simulink model "Simulation_Dual"  (R2022b)
settings: Solver=FixedStepAuto  StartTime=0.0  StopTime=5  FixedStep=1e-6  RelTol=1e-3
model workspace (MAT data in the model file):
  Fbase = 50
  Filter_Ind = 0.00435
  Fs = 10000
  Series1_L = 0.004
  Series2_L = 0.00035
  Shunt_C = 2.2e-06
  Snubber_C = inf
  Snubber_R = 100000
  Ts = 0.0001
  VDCref = 48
undefined symbols (not defined in the file): DiscIntNeverNeededParam, Rdamp, Series1_C, Series2_R
libraries: spsPWMGeneratorDCDCLib x6, spsThreePhaseSeriesRLCBranchLib x6, spsVoltageMeasurementLib x6, spsabctodq0Lib x4, spsThreePhaseVIMeasurementLib x3, spsDCVoltageSourceLib x2, spsdq0toabcLib x2, spsUniversalBridgeLib x2, simulink x1, spspowerguiLib x1
settings Model: Creator=yanni  LastModifiedBy=yanni

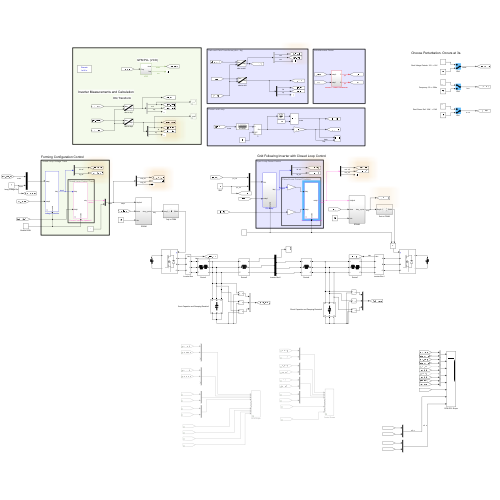
[thumbnail: Simulink's stored preview of the top-level diagram]
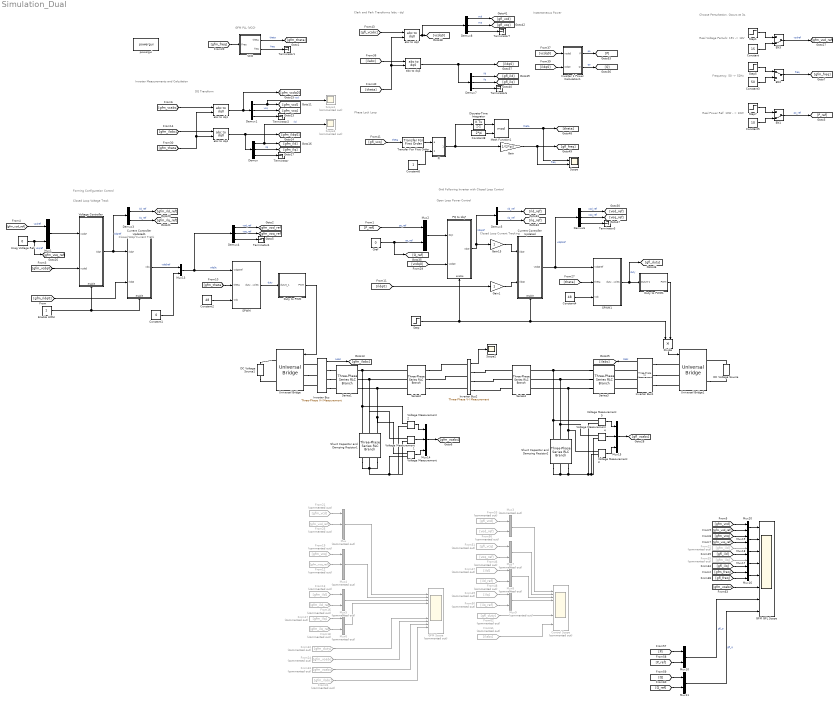
== system Simulation_Dual ==
  note: Closed Loop Voltage Track
  note: Closed Loop Current Track
  note: DQ Transform
  note: GFM PLL (VCO)
  note: Forming Configuration Control
  note: Inverter Measurements and Calculation
  note: Grid Following Inverter with Closed Loop Control
  note: Open Loop Power Control
  note: Closed Loop Current Tracking
  note: Phase Lock Loop
  note: Instantaneous Power
  note: Clark and Park Transforms (abc - dq)
  note: Choose Perturbation. Occurs at 3s.
  note: Real Voltage Perturb: 15V -> 18V
  note: Frequency: 50 -> 52Hz
  note: Real Power Ref: 10W - > 10W
  Constant : Constant  Value=15
  Constant1 : Constant  Value=0
  Constant2 : Constant  Value=48
  Constant3 : Constant  Value=50
  Constant4 : Constant  Value=48
  Constant5 : Constant  Value=10
  Constant6 : Constant
  Constant8 : Constant  Value=2*pi
  Control Scope : Scope  Commented=on  NumInputPorts=12
  Current Controller Updated : Subsystem  mask{Id_Proportional=1.22, Id_Integral=957/16}
      mask prompts: Id_Proportional "Kp"; Id_Integral "Ki"
      settings: PortSchema="{\"entries\":[{\"content\":{\"sides\":[{\"content\":{\"connectorIds\":[\"In1\",\"In2\"]},\"type\":\"ConnectorPlacement.EquallySpacedRectSide\",\"uuid\":\"134caf41-c34b-48d0-a71a-522329c40d8c\"},{\"content\":{\"connectorIds\":[\"Out1\"],\"side\":\"RIGHT\"},\"type\":\"ConnectorPlacement.EquallySpacedRectSide\",\"uuid\":\"de6d8359-09d9-4cb7-8990-bc4b6d48f18d\"},{\"content\":{\"connectorIds\":[],\"side\":\"TOP\"},\"type\":\"ConnectorPlacement.EquallySpacedRectSide\",\"uuid\":\"e2785d07-2ead-4d42-94ac-8025f550e46a\"},{\"content\":{\"connectorIds\":[\"In3\"],\"side\":\"BOTTOM\"},\"type\":\"ConnectorPlacement.EquallySpacedRectSide\",\"uuid\":\"a912a274-012c-4cba-911c-beb79bb7dc91\"}]},\"type\":\"ConnectorPlacement.EquallySpacedConnector\",\"uuid\":\"3c498838-bb9a-4b09-bf48-00f71cabf7b4\"}],\"packageUris\":[\"http://schema.mathworks.com/mf0/Connector/R2020b\"],\"version\":\"1.0\"}"
  Current Controller Updated1 : Subsystem  mask{Id_Proportional=0.61, Id_Integral=240/16}
      mask prompts: Id_Proportional "Kp"; Id_Integral "Ki"
      settings: PortSchema="{\"entries\":[{\"content\":{\"sides\":[{\"content\":{\"connectorIds\":[\"In1\",\"In2\"]},\"type\":\"ConnectorPlacement.EquallySpacedRectSide\",\"uuid\":\"134caf41-c34b-48d0-a71a-522329c40d8c\"},{\"content\":{\"connectorIds\":[\"Out1\"],\"side\":\"RIGHT\"},\"type\":\"ConnectorPlacement.EquallySpacedRectSide\",\"uuid\":\"de6d8359-09d9-4cb7-8990-bc4b6d48f18d\"},{\"content\":{\"connectorIds\":[],\"side\":\"TOP\"},\"type\":\"ConnectorPlacement.EquallySpacedRectSide\",\"uuid\":\"e2785d07-2ead-4d42-94ac-8025f550e46a\"},{\"content\":{\"connectorIds\":[\"In3\"],\"side\":\"BOTTOM\"},\"type\":\"ConnectorPlacement.EquallySpacedRectSide\",\"uuid\":\"a912a274-012c-4cba-911c-beb79bb7dc91\"}]},\"type\":\"ConnectorPlacement.EquallySpacedConnector\",\"uuid\":\"3c498838-bb9a-4b09-bf48-00f71cabf7b4\"}],\"packageUris\":[\"http://schema.mathworks.com/mf0/Connector/R2020b\"],\"version\":\"1.0\"}"
  DC Voltage Source : spsDCVoltageSourceLib/DC Voltage Source  Amplitude=VDCref  Measurements=None
  DC Voltage Source1 : spsDCVoltageSourceLib/DC Voltage Source  Amplitude=48  Measurements=None
  Demux{,1,4,6..8} (6 alike) : Demux  Outputs=3
  Demux3 : Demux  Outputs=2
  Demux5 : Demux  Outputs=2
  Discrete-Time Integrator : DiscreteIntegrator  SampleTime=Ts  ICPrevOutput=DiscIntNeverNeededParam  ICPrevScaledInput=DiscIntNeverNeededParam
  Divide : Product  Inputs=**
  Duty to PWM : Subsystem
  Duty to PWM1 : Subsystem
  EN1 : ManualSwitch  CurrentSetting=0
  EN2 : ManualSwitch
  EN3 : ManualSwitch  CurrentSetting=0
  Enable HIGH : Constant
  From12 : From  Commented=on  GotoTag=gfm_voq_ref
      settings: CloseFcn=tagdialog Close
  From13 : From  Commented=on  GotoTag=gfm_ild
      settings: CloseFcn=tagdialog Close
  From16 : From  Commented=on  GotoTag=gfm_ild_ref
      settings: CloseFcn=tagdialog Close
  From17 : From  Commented=on  GotoTag=gfm_ilq
      settings: CloseFcn=tagdialog Close
  From18 : From  Commented=on  GotoTag=gfm_ilq_ref
      settings: CloseFcn=tagdialog Close
  From19 : From  Commented=on  GotoTag=gfm_vcq
      settings: CloseFcn=tagdialog Close
  From21 : From  Commented=on  GotoTag=gfm_vcd
      settings: CloseFcn=tagdialog Close
  From22 : From  Commented=on  GotoTag=gfm_ild
      settings: CloseFcn=tagdialog Close
  From24 : From  Commented=on  GotoTag=gfm_voabc
      settings: CloseFcn=tagdialog Close
  From25 : From  Commented=on  GotoTag=gfm_vod_ref
      settings: CloseFcn=tagdialog Close
  From31 : From  Commented=on  GotoTag=gfm_ilabc
      settings: CloseFcn=tagdialog Close
  From32 : From  Commented=on  GotoTag=gfm_duty
      settings: CloseFcn=tagdialog Close
  From33 : From  Commented=on  GotoTag=gfm_vcabc
      settings: CloseFcn=tagdialog Close
  From35 : From  Commented=on  GotoTag=gfm_ilq
      settings: CloseFcn=tagdialog Close
  From46 : From  Commented=on  GotoTag=voq_ref
      settings: CloseFcn=tagdialog Close
  From47 : From  Commented=on  GotoTag=ild
      settings: CloseFcn=tagdialog Close
  From48 : From  Commented=on  GotoTag=ild_ref
      settings: CloseFcn=tagdialog Close
  From49 : From  Commented=on  GotoTag=ilq
      settings: CloseFcn=tagdialog Close
  From50 : From  Commented=on  GotoTag=ilq_ref
      settings: CloseFcn=tagdialog Close
  From51 : From  Commented=on  GotoTag=gfl_vcq
      settings: CloseFcn=tagdialog Close
  From53 : From  Commented=on  GotoTag=gfl_vcd
      settings: CloseFcn=tagdialog Close
  From56 : From  Commented=on  GotoTag=vod_ref
      settings: CloseFcn=tagdialog Close
  From61 : From  Commented=on  GotoTag=ilabc
      settings: CloseFcn=tagdialog Close
  From62 : From  Commented=on  GotoTag=gfl_duty
      settings: CloseFcn=tagdialog Close
  GFM GFL Scope : Scope  NumInputPorts=8
  GFM Scope : Scope  Commented=on  NumInputPorts=12
  Gain : Gain  Gain=1/(2*pi)
  Gain1 : Gain
  Gain15 : Gain
  Imag Votlage Ref : Constant  Value=0
  Inverter 1 Power Calculation1 : Subsystem
  Inverter Bus : spsThreePhaseVIMeasurementLib/Three-Phase V-I Measurement  VoltageMeasurement=no  SetLabelV=off  LabelV=Vabc  Vpu=off  VpuLL=off  CurrentMeasurement=yes  SetLabelI=off  LabelI=Iabc  Ipu=off  Pbase=100e6  Vbase=500e3  OutputType=Complex  PhasorSimulation=off  PSBequivalent=0
  Inverter Bus1 : spsThreePhaseVIMeasurementLib/Three-Phase V-I Measurement  VoltageMeasurement=no  SetLabelV=off  LabelV=Vabc  Vpu=off  VpuLL=off  CurrentMeasurement=yes  SetLabelI=off  LabelI=Iabc  Ipu=off  Pbase=100e6  Vbase=500e3  OutputType=Complex  PhasorSimulation=off  PSBequivalent=0
  Inverter Bus2 : spsThreePhaseVIMeasurementLib/Three-Phase V-I Measurement  VoltageMeasurement=phase-to-phase  SetLabelV=off  LabelV=Vabc  Vpu=off  VpuLL=off  CurrentMeasurement=no  SetLabelI=off  LabelI=Iabc  Ipu=off  Pbase=100e6  Vbase=500e3  OutputType=Complex  PhasorSimulation=off  PSBequivalent=0
  Math Function1 : Math  Operator=mod  SignedPower=on
  Mux : Mux  Commented=on  Inputs=3
  Mux{1..2,10..11,13,16..20} (10 alike) : Mux  Inputs=2
  Mux14 : Mux  Inputs=3
  Mux15 : Mux  Inputs=3
  Mux{3,5..9} (6 alike) : Mux  Commented=on  Inputs=2
  Mux4 : Mux  Commented=on  Inputs=3
  PI : Subsystem  mask{Kp_PLL=6.09, Ki_PLL=9.57, IntSat_PLL=20000}
      mask prompts: Kp_PLL "Proportional (P)"; Ki_PLL "Integral (I)"; IntSat_PLL "Integrator Saturation Limit"
      mask DialogControl DescGroupVar Prompt: PLL Parameters
  PQ to Idq* : Subsystem
      settings: PortSchema="{\"entries\":[{\"content\":{\"sides\":[{\"content\":{\"connectorIds\":[\"In1\",\"In2\"]},\"type\":\"ConnectorPlacement.EquallySpacedRectSide\",\"uuid\":\"5271b3ed-46a4-4113-9b69-458d23b85fa2\"},{\"content\":{\"connectorIds\":[\"Out1\"],\"side\":\"RIGHT\"},\"type\":\"ConnectorPlacement.EquallySpacedRectSide\",\"uuid\":\"00fb532b-4b50-4607-a5c4-cd74a5a5fc42\"},{\"content\":{\"connectorIds\":[],\"side\":\"TOP\"},\"type\":\"ConnectorPlacement.EquallySpacedRectSide\",\"uuid\":\"05671b8e-b1fa-45d3-a4a8-1640aa1af326\"},{\"content\":{\"connectorIds\":[\"In3\"],\"side\":\"BOTTOM\"},\"type\":\"ConnectorPlacement.EquallySpacedRectSide\",\"uuid\":\"cfa1ca65-6f63-4245-906b-c8bf76b96ed3\"}]},\"type\":\"ConnectorPlacement.EquallySpacedConnector\",\"uuid\":\"bf062c94-390f-4409-83d1-f8a32d59f496\"}],\"packageUris\":[\"http://schema.mathworks.com/mf0/Connector/R2020b\"],\"version\":\"1.0\"}"
  Qref : Constant  Value=0
  SPWM : Subsystem
  SPWM1 : Subsystem
  Scope : Scope  NumInputPorts=2
  Scope1 : Scope  Commented=on
  Scope2 : Scope
  Scope3 : Scope  Commented=on
  Series1 : spsThreePhaseSeriesRLCBranchLib/Three-Phase Series RLC Branch  LConnTagsString=A|B|C  RConnTagsString=A|B|C  BranchType=RL  Resistance=0.35  Inductance=Series1_L  Capacitance=Series1_C  Measurements=None
  Series2 : spsThreePhaseSeriesRLCBranchLib/Three-Phase Series RLC Branch  LConnTagsString=A|B|C  RConnTagsString=A|B|C  BranchType=L  Resistance=Series2_R  Inductance=Series2_L  Capacitance=1e-6  Measurements=None
  Series3 : spsThreePhaseSeriesRLCBranchLib/Three-Phase Series RLC Branch  LConnTagsString=A|B|C  RConnTagsString=A|B|C  BranchType=RL  Resistance=0.35  Inductance=Series1_L  Capacitance=Series1_C  Measurements=None
  Series4 : spsThreePhaseSeriesRLCBranchLib/Three-Phase Series RLC Branch  LConnTagsString=A|B|C  RConnTagsString=A|B|C  BranchType=L  Resistance=Series2_L  Inductance=Series2_L  Capacitance=1e-6  Measurements=None
  Shunt Capacitor and Damping Resistor1 : spsThreePhaseSeriesRLCBranchLib/Three-Phase Series RLC Branch  LConnTagsString=A|B|C  RConnTagsString=A|B|C  BranchType=C  Resistance=Rdamp  Inductance=1e-3  Capacitance=Shunt_C  Measurements=None
  Shunt Capacitor and Damping Resistor2 : spsThreePhaseSeriesRLCBranchLib/Three-Phase Series RLC Branch  LConnTagsString=A|B|C  RConnTagsString=A|B|C  BranchType=C  Resistance=Rdamp  Inductance=1e-3  Capacitance=Shunt_C  Measurements=None
  Step : Step  SampleTime=0
  Step1 : Step  Time=3  Before=15  After=18
  Step5 : Step  Time=3  Before=50  After=52  SampleTime=0
  Step7 : Step  Time=3  Before=10  After=-10
  Terminator{,1..4,6..7} (7 alike) : Terminator
  Transfer Fcn First Order : simulink/Discrete/Transfer Fcn First Order  PoleZ=exp(-2*pi*100*Ts)  ICPrevOutput=0.0  DoSatur=off
  Universal Bridge : spsUniversalBridgeLib/Universal Bridge  Arms=3  SnubberResistance=Snubber_R  SnubberCapacitance=Snubber_C  Device=MOSFET / Diodes  Ron=1e-3  Lon=0  ForwardVoltages="[  0  0  ]"  ForwardVoltage=0  GTOparameters=[ 10e-6 , 20e-6 ]  IGBTparameters=[ 1e-6 , 2e-6 ]  Measurements=None  Measurements_2=None  converterType=Rectifier
  Universal Bridge1 : spsUniversalBridgeLib/Universal Bridge  Arms=3  SnubberResistance=Snubber_R  SnubberCapacitance=Snubber_C  Device=MOSFET / Diodes  Ron=1e-3  Lon=0  ForwardVoltages="[  0  0  ]"  ForwardVoltage=0  GTOparameters=[ 10e-6 , 20e-6 ]  IGBTparameters=[ 1e-6 , 2e-6 ]  Measurements=All voltages and currents  Measurements_2=None  converterType=Rectifier
  VCO : Subsystem
  Voltage Controller : Subsystem  mask{Id_Proportional=0.028, Id_Integral=8.685*8}
      mask prompts: Id_Proportional "Kp"; Id_Integral "Ki"
      settings: PortSchema="{\"entries\":[{\"content\":{\"sides\":[{\"content\":{\"connectorIds\":[\"In1\",\"In2\"]},\"type\":\"ConnectorPlacement.EquallySpacedRectSide\",\"uuid\":\"134caf41-c34b-48d0-a71a-522329c40d8c\"},{\"content\":{\"connectorIds\":[\"Out1\"],\"side\":\"RIGHT\"},\"type\":\"ConnectorPlacement.EquallySpacedRectSide\",\"uuid\":\"de6d8359-09d9-4cb7-8990-bc4b6d48f18d\"},{\"content\":{\"connectorIds\":[],\"side\":\"TOP\"},\"type\":\"ConnectorPlacement.EquallySpacedRectSide\",\"uuid\":\"e2785d07-2ead-4d42-94ac-8025f550e46a\"},{\"content\":{\"connectorIds\":[\"In3\"],\"side\":\"BOTTOM\"},\"type\":\"ConnectorPlacement.EquallySpacedRectSide\",\"uuid\":\"a912a274-012c-4cba-911c-beb79bb7dc91\"}]},\"type\":\"ConnectorPlacement.EquallySpacedConnector\",\"uuid\":\"3c498838-bb9a-4b09-bf48-00f71cabf7b4\"}],\"packageUris\":[\"http://schema.mathworks.com/mf0/Connector/R2020b\"],\"version\":\"1.0\"}"
  Voltage Measurement{,1..5} (6 alike) : spsVoltageMeasurementLib/Voltage Measurement  PhasorSimulation=off  OutputType=Complex  PSBequivalent=0
  abc to dq{1..4} (4 alike) : spsabctodq0Lib/abc to dq0  Alignment=90 degrees behind phase A axis
  powergui : spspowerguiLib/powergui  Priority=1  SimulationMode=Discrete  SampleTime=1e-6  frequency=60  Iterations=50  frequencyindice=0  Pbase=100e6  ErrMax=1e-4  UnitsV=kV  UnitsW=MW  buscounter=0  FunctionMessages=off  echomessages=off  EnableUseOfTLC=off  CurrentSourceSwitches=off  DisableSnubberDevices=off  DisableRonSwitches=off  DisableVfSwitches=off  DisplayEquations=off  AutomaticDiscreteSolvers=off  SolverType=Tustin/Backward Euler (TBE)  Interpol=off  ExternalGateDelay=off  methode=off  Ts=100  x0status=blocks  SPID=on  SwTol=0  HookPort=off  NonlinearTolerance=1e-4  nMaxIteration=100  ContinueOnMaxIteration=off  RestoreLinks=warning  ResistiveCurrentMeasurement=off  Frange=[0:2:500]  Ylog=off  Xlog=on  ShowGrid=off  save=off  variable=ZData  structure=0  ZoomFFT=off  StartTime=0.0  cycles=1  DisplayStyle=1  fundamental=60  FreqAxis=off  MaxFrequency=1000  frequencyindicesteady=1  RmsSteady=1  display=off
  wires:
  abc to dq1/1 -> [gfm_vcdq0], Demux1/1
  Mux13/1 -> SPWM/1(Vdq0ref), Demux4/1  "vdq0c"
  abc to dq4/1 -> [gfm_ildq0], Demux/1
  [gfm_theta] -> SPWM/2(theta)
  Enable HIGH/1 -> Current Controller Updated1/3(enable), Voltage Controller/3(enable)
  Mux1/1 -> Voltage Controller/1(vsdq*)
  [gfm_vsd_ref] -> Mux1/1  "vsdref"
  Imag Votlage Ref/1 -> [gfm_vsq_ref], Mux1/2  "vsqref"
  Inverter Bus/1 -> [gfm_ilabc]  "iLabc"
  Demux/2 -> [gfm_ilq]  "ilq"
  Demux/1 -> Scope3/1, [gfm_ild]  "ild"
  Demux/3 -> Terminator/1
  Demux3/2 -> [gfm_ilq_ref]  "ilq_ref"
  Demux3/1 -> [gfm_ild_ref]  "ild_ref"
  Demux4/2 -> [gfm_voq_ref]  "voq_ref"
  Demux4/1 -> [gfm_vod_ref]  "vod_ref"
  Demux4/3 -> Terminator4/1
  [gfm_vcdq0] -> Voltage Controller/2(vcdq0)
  [gfm_theta] -> abc to dq1/2, abc to dq4/2
  [gfm_vcabc] -> abc to dq1/1
  Voltage Controller/1(ildq*) -> Current Controller Updated1/1(ildq*), Demux3/1  "ildqref"
  VCO/1(theta) -> [gfm_theta]  "theta"
  VCO/2(freq) -> Terminator1/1  "freq"
  [gfm_ilabc] -> abc to dq4/1
  [gfm_freq] -> VCO/1(Freq)
  Duty to PWM/1(PWM) -> Universal Bridge/1
  From25/1 -> Mux/2
  From17/1 -> Mux6/1
  Mux/1 -> GFM Scope/1
  From33/1 -> GFM Scope/11
  From32/1 -> GFM Scope/9
  From12/1 -> Mux4/2
  Mux4/1 -> GFM Scope/2
  From21/1 -> Mux/1
  Mux5/1 -> GFM Scope/3
  From31/1 -> GFM Scope/12
  Mux6/1 -> GFM Scope/4
  From24/1 -> GFM Scope/10
  From16/1 -> Mux5/2
  From13/1 -> Mux5/1
  From18/1 -> Mux6/2
  From19/1 -> Mux4/1
  Demux1/2 -> [gfm_vcq]  "vcq"
  Demux1/1 -> Scope1/1, [gfm_vcd]  "vcd"
  Demux1/3 -> Terminator2/1
  Inverter Bus1/1 -> [ilabc]  "ilabc"
  [ildq0] -> Gain1/1
  SPWM1/1(duty_cycles) -> [gfl_duty], Duty to PWM1/1(Duty0-1)  "duty"
  Mux2/1 -> PQ to Idq*/1(PQ*)
  [vcdq0] -> PQ to Idq*/2(vodq0)
  [P_ref] -> Mux2/1  "po_ref"
  Current Controller Updated/1(vtdq0) -> SPWM1/1(Vdq0ref), Demux6/1  "vdq0ref"
  Demux6/1 -> [vod_ref]  "vod_ref"
  [theta] -> SPWM1/2(theta)
  Demux5/2 -> [ilq_ref]  "ilq_ref"
  PQ to Idq*/1(iIdq*) -> Demux5/1, Gain15/1  "ildqref"
  Demux6/3 -> Terminator3/1
  Demux5/1 -> [ild_ref]  "ild_ref"
  Demux6/2 -> [voq_ref]  "voq_ref"
  Qref/1 -> [Q_ref], Mux2/2  "qo_ref"
  Step/1 -> PQ to Idq*/3(enable), Divide/1, Current Controller Updated/3(enable)
  Gain15/1 -> Current Controller Updated/1(ildq*)
  Constant8/1 -> Math Function1/2
  Gain/1 -> [gfl_freq], Scope/2  "freq"
  Discrete-Time Integrator/1 -> Math Function1/1
  Math Function1/1 -> [theta], Scope/1  "theta"
  PI/1(Out) -> Gain/1, Discrete-Time Integrator/1
  Inverter 1 Power Calculation1/2(Q) -> [Q]  "qo"
  [vcdq0] -> Inverter 1 Power Calculation1/1(vodq0)
  Inverter 1 Power Calculation1/1(P) -> [P]  "po"
  [ildq0] -> Inverter 1 Power Calculation1/2(iodq0)
  From61/1 -> Control Scope/12
  Mux8/1 -> Control Scope/3
  From46/1 -> Mux7/2
  [Q] -> Mux11/1
  From51/1 -> Mux7/1
  Mux3/1 -> Control Scope/1
  From48/1 -> Mux8/2
  Mux7/1 -> Control Scope/2
  Mux9/1 -> Control Scope/4
  From53/1 -> Mux3/1
  [Q_ref] -> Mux11/2
  [P] -> Mux10/1
  From62/1 -> Control Scope/9
  From47/1 -> Mux8/1
  From50/1 -> Mux9/2
  From49/1 -> Mux9/1
  From56/1 -> Mux3/2
  [P_ref] -> Mux10/2
  [gfm_vcabc] -> GFM GFL Scope/6
  Gain1/1 -> Current Controller Updated/2(ildq0)
  [gfl_vcq] -> Transfer Fcn First Order/1  "theta"
  Demux7/3 -> Terminator6/1
  Demux7/2 -> [gfl_ilq]  "ilq"
  Demux7/1 -> [gfl_ild]  "ild"
  Demux8/1 -> [gfl_vcd]  "vcd"
  Demux8/3 -> Terminator7/1
  abc to dq3/1 -> Demux7/1, [ildq0]
  [gfl_vcabc] -> abc to dq2/1
  Demux8/2 -> [gfl_vcq]  "vcq"
  [ilabc] -> abc to dq3/1
  [theta] -> abc to dq3/2, abc to dq2/2
  abc to dq2/1 -> Demux8/1, [vcdq0]
  Constant1/1 -> Mux13/2
  Constant2/1 -> SPWM/3(Vdc)
  SPWM/1(duty_cycles) -> Duty to PWM/1(duty0_1)  "duty"
  Constant4/1 -> SPWM1/3(Vdc)
  Voltage Measurement/1 -> Mux14/3
  Voltage Measurement1/1 -> Mux14/2
  Mux14/1 -> [gfm_vcabc]
  Voltage Measurement2/1 -> Mux14/1
  Mux15/1 -> [gfl_vcabc]
  Voltage Measurement4/1 -> Mux15/2
  Voltage Measurement5/1 -> Mux15/1
  Voltage Measurement3/1 -> Mux15/3
  Current Controller Updated1/1(vdq) -> Mux13/1  "vdq0ref"
  [gfm_ildq0] -> Current Controller Updated1/2(ildq0)
  Inverter Bus2/1 -> Scope2/1
  Divide/1 -> Universal Bridge1/1
  Duty to PWM1/1(PWM) -> Divide/2
  Mux18/1 -> GFM GFL Scope/3
  From35/1 -> Mux17/1
  [gfl_ilq] -> Mux17/2
  Mux16/1 -> GFM GFL Scope/5
  Mux20/1 -> GFM GFL Scope/1
  Mux17/1 -> GFM GFL Scope/4
  Mux19/1 -> GFM GFL Scope/2
  Mux11/1 -> GFM GFL Scope/8  "gfl_q"
  [gfl_freq] -> Mux16/2
  [gfl_ild] -> Mux18/2
  [gfm_freq] -> Mux16/1
  [gfm_vcd] -> Mux20/1
  From22/1 -> Mux18/1
  [gfm_vcq] -> Mux19/1
  Mux10/1 -> GFM GFL Scope/7  "gfl_p"
  [gfm_vsd_ref] -> Mux20/2
  [gfm_vsq_ref] -> Mux19/2
  EN2/1 -> [gfm_freq]  "freq"
  EN1/1 -> [P_ref]  "po_ref"
  Step1/1 -> EN3/1
  Step7/1 -> EN1/1
  Step5/1 -> EN2/1
  Constant/1 -> EN3/2
  Constant3/1 -> EN2/2
  Constant5/1 -> EN1/2
  EN3/1 -> [gfm_vsd_ref]  "vsdref"
  Transfer Fcn First Order/1 -> PI/1(e)
  Constant6/1 -> PI/2(RST)
  connections:
  DC Voltage Source1/LConn1 -- Universal Bridge/RConn2
  Universal Bridge/RConn1 -- DC Voltage Source1/RConn1
  Series1/RConn1 -- Series2/LConn1 -- Shunt Capacitor and Damping Resistor1/LConn1 -- Voltage Measurement2/LConn1
  Series1/RConn3 -- Series2/LConn3 -- Shunt Capacitor and Damping Resistor1/LConn3 -- Voltage Measurement/LConn1
  Inverter Bus/RConn2 -- Series1/LConn2
  Inverter Bus/RConn1 -- Series1/LConn1
  Inverter Bus/RConn3 -- Series1/LConn3
  Inverter Bus/LConn1 -- Universal Bridge/LConn1
  Universal Bridge/LConn2 -- Inverter Bus/LConn2
  Inverter Bus/LConn3 -- Universal Bridge/LConn3
  Shunt Capacitor and Damping Resistor2/LConn2 -- Series3/RConn2 -- Series4/LConn2 -- Voltage Measurement4/LConn1
  Shunt Capacitor and Damping Resistor2/LConn3 -- Series3/RConn3 -- Series4/LConn3 -- Voltage Measurement3/LConn1
  Shunt Capacitor and Damping Resistor2/LConn1 -- Series3/RConn1 -- Series4/LConn1 -- Voltage Measurement5/LConn1
  DC Voltage Source/RConn1 -- Universal Bridge1/RConn1
  Inverter Bus1/RConn2 -- Series3/LConn2
  Inverter Bus1/RConn3 -- Series3/LConn3
  Inverter Bus1/LConn1 -- Universal Bridge1/LConn1
  Inverter Bus1/RConn1 -- Series3/LConn1
  Inverter Bus1/LConn2 -- Universal Bridge1/LConn2
  Inverter Bus1/LConn3 -- Universal Bridge1/LConn3
  Universal Bridge1/RConn2 -- DC Voltage Source/LConn1
  Voltage Measurement/LConn2 -- Shunt Capacitor and Damping Resistor1/RConn1 -- Shunt Capacitor and Damping Resistor1/RConn3 -- Shunt Capacitor and Damping Resistor1/RConn2 -- Voltage Measurement2/LConn2 -- Voltage Measurement1/LConn2
  Voltage Measurement3/LConn2 -- Voltage Measurement4/LConn2 -- Voltage Measurement5/LConn2 -- Shunt Capacitor and Damping Resistor2/RConn1 -- Shunt Capacitor and Damping Resistor2/RConn2 -- Shunt Capacitor and Damping Resistor2/RConn3
  Series1/RConn2 -- Series2/LConn2 -- Voltage Measurement1/LConn1 -- Shunt Capacitor and Damping Resistor1/LConn2
  Series2/RConn1 -- Inverter Bus2/LConn1
  Series2/RConn2 -- Inverter Bus2/LConn2
  Series2/RConn3 -- Inverter Bus2/LConn3
  Inverter Bus2/RConn3 -- Series4/RConn3
  Inverter Bus2/RConn1 -- Series4/RConn1
  Inverter Bus2/RConn2 -- Series4/RConn2

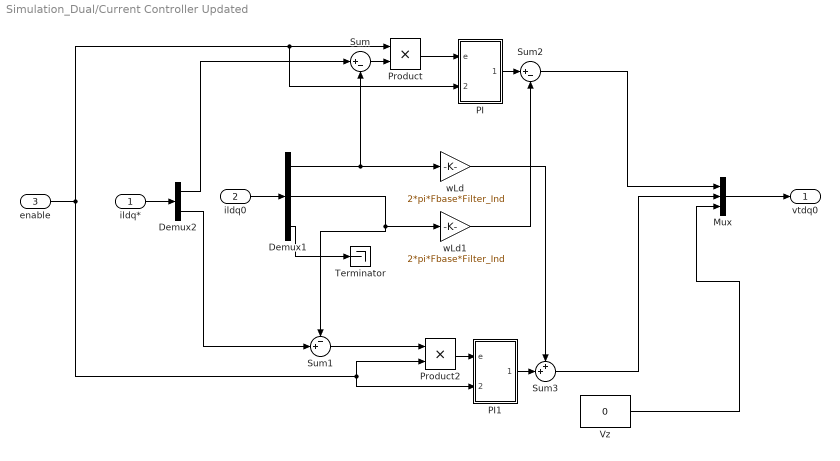
== system Simulation_Dual/Current Controller Updated ==
  ildq* : Inport
  ildq0 : Inport  Port=2
  enable : Inport  Port=3
  Demux1 : Demux  Outputs=3
  Demux2 : Demux  Outputs=2
  Mux : Mux  Inputs=3
  PI : Subsystem
  PI1 : Subsystem
  Product : Product  RndMeth=Zero
  Product2 : Product  RndMeth=Zero
  Sum : Sum  Inputs=|+-
  Sum1 : Sum  Inputs=-+|
  Sum2 : Sum  Inputs=|+-
  Sum3 : Sum  Inputs=++|
  Terminator : Terminator
  Vz : Constant  Value=0
  wLd : Gain  Gain=2*pi*Fbase*Filter_Ind
  wLd1 : Gain  Gain=2*pi*Fbase*Filter_Ind
  vtdq0 : Outport
  wires:
  Sum2/1 -> Mux/1
  Sum3/1 -> Mux/2
  ildq0/1 -> Demux1/1
  Mux/1 -> vtdq0/1
  Demux1/3 -> Terminator/1
  ildq*/1 -> Demux2/1
  Demux2/1 -> Sum/1
  Demux2/2 -> Sum1/2
  Product/1 -> PI/1(e)
  Sum1/1 -> Product2/1
  PI/1(Out) -> Sum2/1
  wLd/1 -> Sum3/1
  wLd1/1 -> Sum2/2
  PI1/1(Out) -> Sum3/2
  Demux1/2 -> Sum1/1, wLd1/1
  Demux1/1 -> wLd/1, Sum/2
  Product2/1 -> PI1/1(e)
  Sum/1 -> Product/2
  enable/1 -> Product/1, PI/2(RST), PI1/2(RST), Product2/2
  Vz/1 -> Mux/3

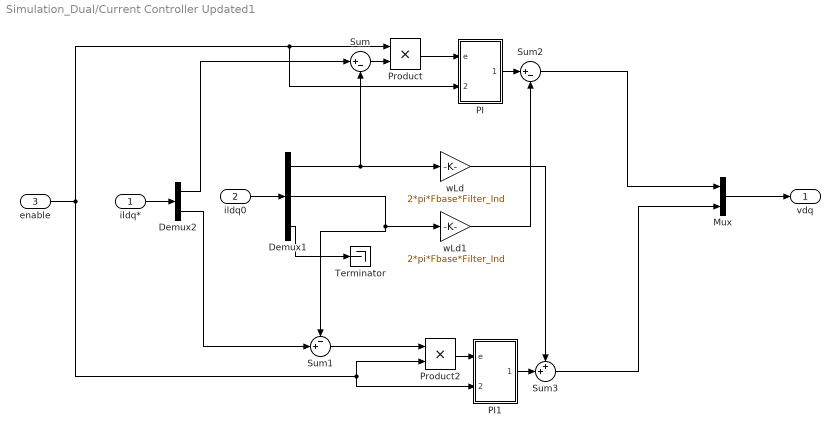
== system Simulation_Dual/Current Controller Updated1 ==
  ildq* : Inport
  ildq0 : Inport  Port=2
  enable : Inport  Port=3
  Demux1 : Demux  Outputs=3
  Demux2 : Demux  Outputs=2
  Mux : Mux  Inputs=2
  PI : Subsystem
  PI1 : Subsystem
  Product : Product  RndMeth=Zero
  Product2 : Product  RndMeth=Zero
  Sum : Sum  Inputs=|+-
  Sum1 : Sum  Inputs=-+|
  Sum2 : Sum  Inputs=|+-
  Sum3 : Sum  Inputs=++|
  Terminator : Terminator
  wLd : Gain  Gain=2*pi*Fbase*Filter_Ind
  wLd1 : Gain  Gain=2*pi*Fbase*Filter_Ind
  vdq : Outport
  wires:
  Sum2/1 -> Mux/1
  Sum3/1 -> Mux/2
  ildq0/1 -> Demux1/1
  Mux/1 -> vdq/1
  Demux1/3 -> Terminator/1
  ildq*/1 -> Demux2/1
  Demux2/1 -> Sum/1
  Demux2/2 -> Sum1/2
  Product/1 -> PI/1(e)
  Sum1/1 -> Product2/1
  PI/1(Out) -> Sum2/1
  wLd/1 -> Sum3/1
  wLd1/1 -> Sum2/2
  PI1/1(Out) -> Sum3/2
  Demux1/2 -> Sum1/1, wLd1/1
  Demux1/1 -> wLd/1, Sum/2
  Product2/1 -> PI1/1(e)
  Sum/1 -> Product/2
  enable/1 -> Product/1, PI/2(RST), PI1/2(RST), Product2/2

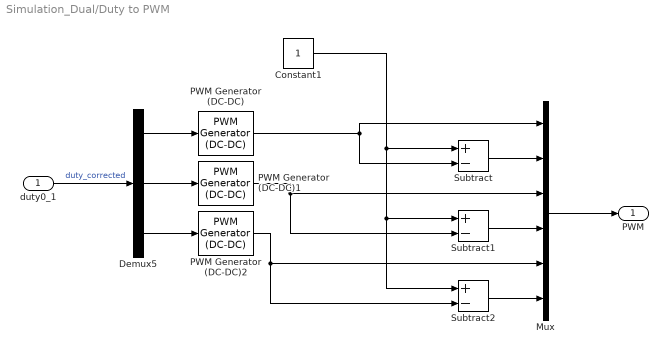
== system Simulation_Dual/Duty to PWM ==
  duty0_1 : Inport
  Constant1 : Constant
  Demux5 : Demux  Outputs=3
  Mux : Mux  Inputs=6
  PWM Generator (DC-DC) : spsPWMGeneratorDCDCLib/PWM Generator (DC-DC)  Fsw=Fs  Ts=0
  PWM Generator (DC-DC)1 : spsPWMGeneratorDCDCLib/PWM Generator (DC-DC)  Fsw=Fs  Ts=0
  PWM Generator (DC-DC)2 : spsPWMGeneratorDCDCLib/PWM Generator (DC-DC)  Fsw=Fs  Ts=0
  Subtract : Sum  Inputs=+-
  Subtract1 : Sum  Inputs=+-
  Subtract2 : Sum  Inputs=+-
  PWM : Outport
  wires:
  PWM Generator (DC-DC)1/1 -> Subtract1/2, Mux/3
  Demux5/2 -> PWM Generator (DC-DC)1/1
  Demux5/1 -> PWM Generator (DC-DC)/1
  Demux5/3 -> PWM Generator (DC-DC)2/1
  PWM Generator (DC-DC)2/1 -> Subtract2/2, Mux/5
  duty0_1/1 -> Demux5/1  "duty_corrected"
  Subtract1/1 -> Mux/4
  Subtract2/1 -> Mux/6
  PWM Generator (DC-DC)/1 -> Mux/1, Subtract/2
  Constant1/1 -> Subtract2/1, Subtract1/1, Subtract/1
  Subtract/1 -> Mux/2
  Mux/1 -> PWM/1

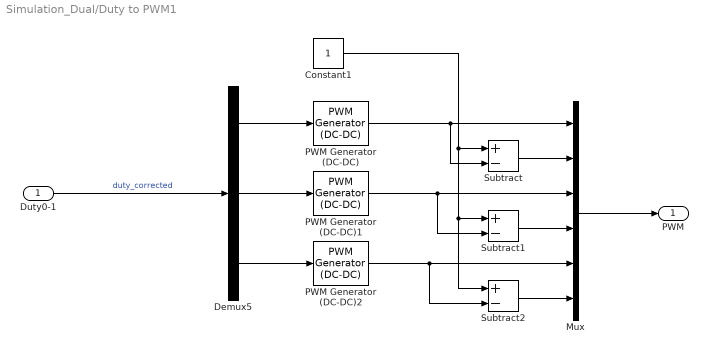
== system Simulation_Dual/Duty to PWM1 ==
  Duty0-1 : Inport
  Constant1 : Constant
  Demux5 : Demux  Outputs=3
  Mux : Mux  Inputs=6
  PWM Generator (DC-DC) : spsPWMGeneratorDCDCLib/PWM Generator (DC-DC)  Fsw=Fs  Ts=0
  PWM Generator (DC-DC)1 : spsPWMGeneratorDCDCLib/PWM Generator (DC-DC)  Fsw=Fs  Ts=0
  PWM Generator (DC-DC)2 : spsPWMGeneratorDCDCLib/PWM Generator (DC-DC)  Fsw=Fs  Ts=0
  Subtract : Sum  Inputs=+-
  Subtract1 : Sum  Inputs=+-
  Subtract2 : Sum  Inputs=+-
  PWM : Outport
  wires:
  Demux5/1 -> PWM Generator (DC-DC)/1
  PWM Generator (DC-DC)2/1 -> Subtract2/2, Mux/5
  Subtract1/1 -> Mux/4
  Demux5/3 -> PWM Generator (DC-DC)2/1
  Duty0-1/1 -> Demux5/1  "duty_corrected"
  Constant1/1 -> Subtract2/1, Subtract1/1, Subtract/1
  Demux5/2 -> PWM Generator (DC-DC)1/1
  Subtract2/1 -> Mux/6
  PWM Generator (DC-DC)1/1 -> Subtract1/2, Mux/3
  PWM Generator (DC-DC)/1 -> Subtract/2, Mux/1
  Subtract/1 -> Mux/2
  Mux/1 -> PWM/1

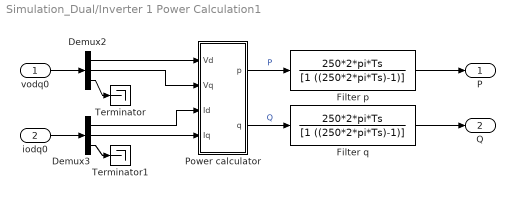
== system Simulation_Dual/Inverter 1 Power Calculation1 ==
  vodq0 : Inport
  iodq0 : Inport  Port=2
  Demux2 : Demux  Outputs=3
  Demux3 : Demux  Outputs=3
  Filter p : DiscreteTransferFcn  Numerator=250*2*pi*Ts  Denominator=[1 ((250*2*pi*Ts)-1)]  SampleTime=Ts
  Filter q : DiscreteTransferFcn  Numerator=250*2*pi*Ts  Denominator=[1 ((250*2*pi*Ts)-1)]  SampleTime=Ts
  Power calculator : Subsystem
  Terminator : Terminator
  Terminator1 : Terminator
  P : Outport
  Q : Outport  Port=2
  wires:
  vodq0/1 -> Demux2/1
  Demux2/1 -> Power calculator/1(Vd)
  Demux2/2 -> Power calculator/2(Vq)
  Demux3/1 -> Power calculator/3(Id)
  Demux3/2 -> Power calculator/4(Iq)
  iodq0/1 -> Demux3/1
  Power calculator/1(p) -> Filter p/1  "P"
  Power calculator/2(q) -> Filter q/1  "Q"
  Demux2/3 -> Terminator/1
  Demux3/3 -> Terminator1/1
  Filter p/1 -> P/1
  Filter q/1 -> Q/1

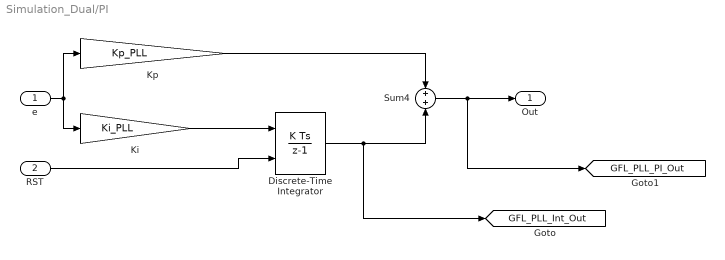
== system Simulation_Dual/PI ==
  e : Inport
  RST : Inport  Port=2
  Discrete-Time Integrator : DiscreteIntegrator  gainval=1  ExternalReset=either  InitialCondition=2*pi*Fbase  SampleTime=Ts  LimitOutput=on  UpperSaturationLimit=2*pi*Fbase + IntSat_PLL  LowerSaturationLimit=2*pi*Fbase - IntSat_PLL  ICPrevOutput=DiscIntNeverNeededParam  ICPrevScaledInput=DiscIntNeverNeededParam
  Ki : Gain  Gain=Ki_PLL  SaturateOnIntegerOverflow=on  OutDataTypeStr=Inherit: Same as input  ParamDataTypeStr=Inherit: Same as input
  Kp : Gain  Gain=Kp_PLL  SaturateOnIntegerOverflow=on  OutDataTypeStr=Inherit: Same as input  ParamDataTypeStr=Inherit: Same as input
  Sum4 : Sum  SaturateOnIntegerOverflow=on
  Out : Outport
  tag scope: GFL_PLL_Int_Out=global, GFL_PLL_PI_Out=global
  wires:
  Ki/1 -> Discrete-Time Integrator/1
  Kp/1 -> Sum4/1
  e/1 -> Ki/1, Kp/1
  RST/1 -> Discrete-Time Integrator/2
  Discrete-Time Integrator/1 -> [GFL_PLL_Int_Out], Sum4/2
  Sum4/1 -> [GFL_PLL_PI_Out], Out/1

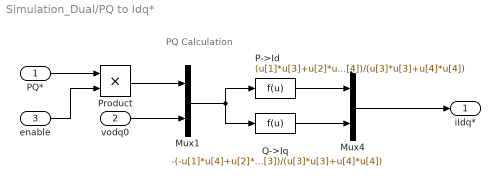
== system Simulation_Dual/PQ to Idq* ==
  note: PQ Calculation
  PQ* : Inport
  vodq0 : Inport  Port=2
  enable : Inport  Port=3
  Mux1 : Mux  Inputs=2
  Mux4 : Mux  Inputs=2
  P->Id : Fcn  Expr=(u[1]*u[3]+u[2]*u[4])/(u[3]*u[3]+u[4]*u[4])
  Product : Product  RndMeth=Zero
  Q->Iq : Fcn  Expr=-(-u[1]*u[4]+u[2]*u[3])/(u[3]*u[3]+u[4]*u[4])
  iIdq* : Outport
  wires:
  enable/1 -> Product/2
  Product/1 -> Mux1/1
  Mux1/1 -> P->Id/1, Q->Iq/1
  P->Id/1 -> Mux4/1
  Q->Iq/1 -> Mux4/2
  Mux4/1 -> iIdq*/1
  vodq0/1 -> Mux1/2
  PQ*/1 -> Product/1

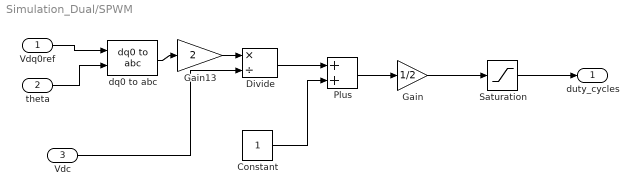
== system Simulation_Dual/SPWM ==
  Vdq0ref : Inport
  theta : Inport  Port=2
  Vdc : Inport  Port=3
  Constant : Constant
  Divide : Product  Inputs=*/
  Gain : Gain  Gain=1/2
  Gain13 : Gain  Gain=2
  Plus : Sum
  Saturation : Saturate  UpperLimit=0.9  LowerLimit=0.1
  dq0 to abc : spsdq0toabcLib/dq0 to abc  Alignment=90 degrees behind phase A axis
  duty_cycles : Outport
  wires:
  Vdq0ref/1 -> dq0 to abc/1
  Gain/1 -> Saturation/1
  theta/1 -> dq0 to abc/2
  Constant/1 -> Plus/2
  Plus/1 -> Gain/1
  Saturation/1 -> duty_cycles/1
  dq0 to abc/1 -> Gain13/1
  Gain13/1 -> Divide/1
  Vdc/1 -> Divide/2
  Divide/1 -> Plus/1

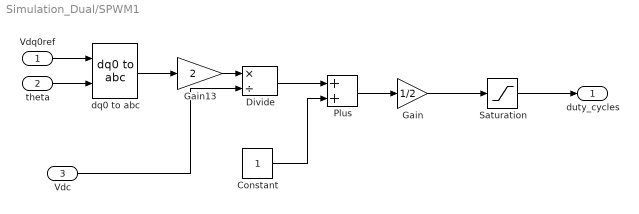
== system Simulation_Dual/SPWM1 ==
  Vdq0ref : Inport
  theta : Inport  Port=2
  Vdc : Inport  Port=3
  Constant : Constant
  Divide : Product  Inputs=*/
  Gain : Gain  Gain=1/2
  Gain13 : Gain  Gain=2
  Plus : Sum
  Saturation : Saturate  UpperLimit=0.9  LowerLimit=0.1
  dq0 to abc : spsdq0toabcLib/dq0 to abc  Alignment=90 degrees behind phase A axis
  duty_cycles : Outport
  wires:
  Vdq0ref/1 -> dq0 to abc/1
  Gain/1 -> Saturation/1
  theta/1 -> dq0 to abc/2
  Constant/1 -> Plus/2
  Plus/1 -> Gain/1
  Saturation/1 -> duty_cycles/1
  dq0 to abc/1 -> Gain13/1
  Gain13/1 -> Divide/1
  Vdc/1 -> Divide/2
  Divide/1 -> Plus/1

== system Simulation_Dual/VCO ==
  Freq : Inport
  Constant2 : Constant  Value=2*pi
  Discrete-Time Integrator : DiscreteIntegrator  SampleTime=Ts  ICPrevOutput=DiscIntNeverNeededParam  ICPrevScaledInput=DiscIntNeverNeededParam
  Gain : Gain  Gain=2*pi
  Math Function1 : Math  Operator=mod  SignedPower=on
  theta : Outport
  freq : Outport  Port=2
  wires:
  Constant2/1 -> Math Function1/2
  Discrete-Time Integrator/1 -> Math Function1/1
  Math Function1/1 -> theta/1
  Freq/1 -> Gain/1, freq/1
  Gain/1 -> Discrete-Time Integrator/1

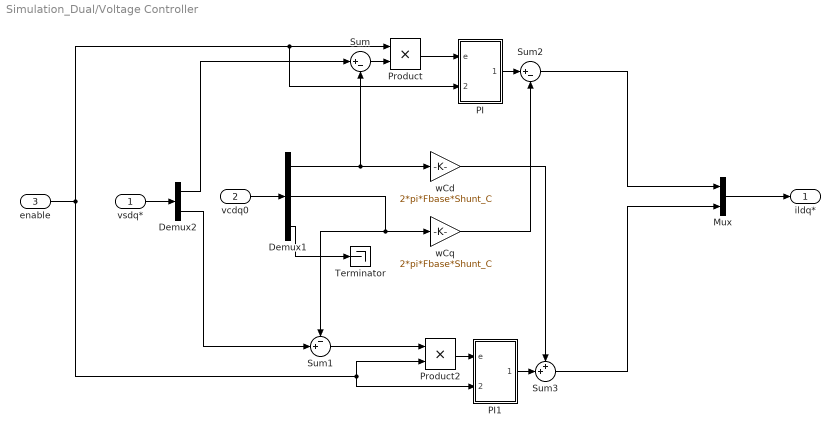
== system Simulation_Dual/Voltage Controller ==
  vsdq* : Inport
  vcdq0 : Inport  Port=2
  enable : Inport  Port=3
  Demux1 : Demux  Outputs=3
  Demux2 : Demux  Outputs=2
  Mux : Mux  Inputs=2
  PI : Subsystem
  PI1 : Subsystem
  Product : Product  RndMeth=Zero
  Product2 : Product  RndMeth=Zero
  Sum : Sum  Inputs=|+-
  Sum1 : Sum  Inputs=-+|
  Sum2 : Sum  Inputs=|+-
  Sum3 : Sum  Inputs=++|
  Terminator : Terminator
  wCd : Gain  Gain=2*pi*Fbase*Shunt_C
  wCq : Gain  Gain=2*pi*Fbase*Shunt_C
  ildq* : Outport
  wires:
  Sum2/1 -> Mux/1
  Sum3/1 -> Mux/2
  vcdq0/1 -> Demux1/1
  Mux/1 -> ildq*/1
  Demux1/3 -> Terminator/1
  vsdq*/1 -> Demux2/1
  Demux2/1 -> Sum/1
  Demux2/2 -> Sum1/2
  Product/1 -> PI/1(e)
  Sum1/1 -> Product2/1
  PI/1(Out) -> Sum2/1
  wCd/1 -> Sum3/1
  wCq/1 -> Sum2/2
  PI1/1(Out) -> Sum3/2
  Demux1/2 -> Sum1/1, wCq/1
  Demux1/1 -> wCd/1, Sum/2
  Product2/1 -> PI1/1(e)
  Sum/1 -> Product/2
  enable/1 -> Product/1, PI/2(RST), PI1/2(RST), Product2/2

== system Simulation_Dual/Current Controller Updated/PI ==
  e : Inport
  RST : Inport  Port=2
  Discrete-Time Integrator : DiscreteIntegrator  gainval=1  ExternalReset=either  SampleTime=Ts  LimitOutput=on  UpperSaturationLimit=20000  LowerSaturationLimit=-20000  ICPrevOutput=DiscIntNeverNeededParam  ICPrevScaledInput=DiscIntNeverNeededParam
  Ki : Gain  Gain=Id_Integral  SaturateOnIntegerOverflow=on  OutDataTypeStr=Inherit: Same as input  ParamDataTypeStr=Inherit: Same as input
  Kp : Gain  Gain=Id_Proportional  SaturateOnIntegerOverflow=on  OutDataTypeStr=Inherit: Same as input  ParamDataTypeStr=Inherit: Same as input
  Sum4 : Sum  SaturateOnIntegerOverflow=on
  Out : Outport
  wires:
  Ki/1 -> Discrete-Time Integrator/1
  Kp/1 -> Sum4/1
  e/1 -> Ki/1, Kp/1
  Discrete-Time Integrator/1 -> Sum4/2
  Sum4/1 -> Out/1
  RST/1 -> Discrete-Time Integrator/2

== system Simulation_Dual/Current Controller Updated/PI1 ==
  e : Inport
  RST : Inport  Port=2
  Discrete-Time Integrator : DiscreteIntegrator  gainval=1  ExternalReset=either  SampleTime=Ts  LimitOutput=on  UpperSaturationLimit=20000  LowerSaturationLimit=-20000  ICPrevOutput=DiscIntNeverNeededParam  ICPrevScaledInput=DiscIntNeverNeededParam
  Ki : Gain  Gain=Id_Integral  SaturateOnIntegerOverflow=on  OutDataTypeStr=Inherit: Same as input  ParamDataTypeStr=Inherit: Same as input
  Kp : Gain  Gain=Id_Proportional  SaturateOnIntegerOverflow=on  OutDataTypeStr=Inherit: Same as input  ParamDataTypeStr=Inherit: Same as input
  Sum4 : Sum  SaturateOnIntegerOverflow=on
  Out : Outport
  wires:
  Ki/1 -> Discrete-Time Integrator/1
  Kp/1 -> Sum4/1
  e/1 -> Ki/1, Kp/1
  Discrete-Time Integrator/1 -> Sum4/2
  Sum4/1 -> Out/1
  RST/1 -> Discrete-Time Integrator/2

== system Simulation_Dual/Current Controller Updated1/PI ==
  e : Inport
  RST : Inport  Port=2
  Discrete-Time Integrator : DiscreteIntegrator  gainval=1  ExternalReset=either  SampleTime=Ts  LimitOutput=on  UpperSaturationLimit=20000  LowerSaturationLimit=-20000  ICPrevOutput=DiscIntNeverNeededParam  ICPrevScaledInput=DiscIntNeverNeededParam
  Ki : Gain  Gain=Id_Integral  SaturateOnIntegerOverflow=on  OutDataTypeStr=Inherit: Same as input  ParamDataTypeStr=Inherit: Same as input
  Kp : Gain  Gain=Id_Proportional  SaturateOnIntegerOverflow=on  OutDataTypeStr=Inherit: Same as input  ParamDataTypeStr=Inherit: Same as input
  Sum4 : Sum  SaturateOnIntegerOverflow=on
  Out : Outport
  wires:
  Ki/1 -> Discrete-Time Integrator/1
  Kp/1 -> Sum4/1
  e/1 -> Ki/1, Kp/1
  Discrete-Time Integrator/1 -> Sum4/2
  Sum4/1 -> Out/1
  RST/1 -> Discrete-Time Integrator/2

== system Simulation_Dual/Current Controller Updated1/PI1 ==
  e : Inport
  RST : Inport  Port=2
  Discrete-Time Integrator : DiscreteIntegrator  gainval=1  ExternalReset=either  SampleTime=Ts  LimitOutput=on  UpperSaturationLimit=20000  LowerSaturationLimit=-20000  ICPrevOutput=DiscIntNeverNeededParam  ICPrevScaledInput=DiscIntNeverNeededParam
  Ki : Gain  Gain=Id_Integral  SaturateOnIntegerOverflow=on  OutDataTypeStr=Inherit: Same as input  ParamDataTypeStr=Inherit: Same as input
  Kp : Gain  Gain=Id_Proportional  SaturateOnIntegerOverflow=on  OutDataTypeStr=Inherit: Same as input  ParamDataTypeStr=Inherit: Same as input
  Sum4 : Sum  SaturateOnIntegerOverflow=on
  Out : Outport
  wires:
  Ki/1 -> Discrete-Time Integrator/1
  Kp/1 -> Sum4/1
  e/1 -> Ki/1, Kp/1
  Discrete-Time Integrator/1 -> Sum4/2
  Sum4/1 -> Out/1
  RST/1 -> Discrete-Time Integrator/2

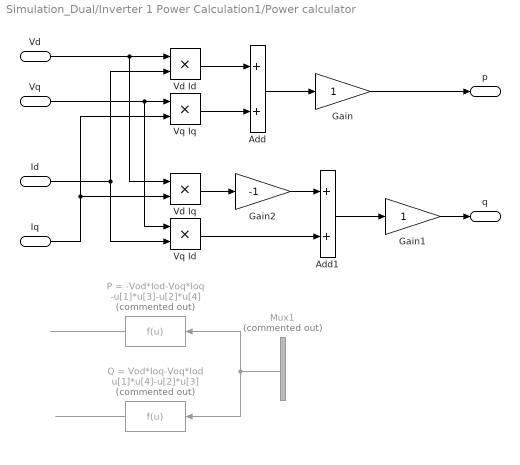
== system Simulation_Dual/Inverter 1 Power Calculation1/Power calculator ==
  Vd : Inport
  Vq : Inport  Port=2
  Id : Inport  Port=3
  Iq : Inport  Port=4
  Add : Sum
  Add1 : Sum
  Gain : Gain
  Gain1 : Gain
  Gain2 : Gain  Gain=-1
  Mux1 : Mux  Commented=on
  P = -Vod*Iod-Voq*Ioq : Fcn  Commented=on  Expr=-u[1]*u[3]-u[2]*u[4]
  Q = Vod*Ioq-Voq*Iod : Fcn  Commented=on  Expr=u[1]*u[4]-u[2]*u[3]
  Vd Id : Product
  Vd Iq : Product
  Vq Id : Product
  Vq Iq : Product
  p : Outport
  q : Outport  Port=2
  wires:
  Q = Vod*Ioq-Voq*Iod/1 -> ?
  P = -Vod*Iod-Voq*Ioq/1 -> ?
  Mux1/1 -> Q = Vod*Ioq-Voq*Iod/1, P = -Vod*Iod-Voq*Ioq/1
  Gain/1 -> p/1
  Add/1 -> Gain/1
  Add1/1 -> Gain1/1
  Gain1/1 -> q/1
  Vd Id/1 -> Add/1
  Vq Iq/1 -> Add/2
  Vq Id/1 -> Add1/2
  Vd Iq/1 -> Gain2/1
  Vd/1 -> Vd Iq/1, Vd Id/1
  Id/1 -> Vd Id/2, Vq Id/2
  Vq/1 -> Vq Id/1, Vq Iq/1
  Iq/1 -> Vd Iq/2, Vq Iq/2
  Gain2/1 -> Add1/1

== system Simulation_Dual/Voltage Controller/PI ==
  e : Inport
  RST : Inport  Port=2
  Discrete-Time Integrator : DiscreteIntegrator  gainval=1  ExternalReset=either  SampleTime=Ts  LimitOutput=on  UpperSaturationLimit=2000  LowerSaturationLimit=-2000  ICPrevOutput=DiscIntNeverNeededParam  ICPrevScaledInput=DiscIntNeverNeededParam
  Ki : Gain  Gain=Id_Integral  SaturateOnIntegerOverflow=on  OutDataTypeStr=Inherit: Same as input  ParamDataTypeStr=Inherit: Same as input
  Kp : Gain  Gain=Id_Proportional  SaturateOnIntegerOverflow=on  OutDataTypeStr=Inherit: Same as input  ParamDataTypeStr=Inherit: Same as input
  Sum4 : Sum  SaturateOnIntegerOverflow=on
  Out : Outport
  wires:
  Ki/1 -> Discrete-Time Integrator/1
  Kp/1 -> Sum4/1
  e/1 -> Ki/1, Kp/1
  Discrete-Time Integrator/1 -> Sum4/2
  Sum4/1 -> Out/1
  RST/1 -> Discrete-Time Integrator/2

== system Simulation_Dual/Voltage Controller/PI1 ==
  e : Inport
  RST : Inport  Port=2
  Discrete-Time Integrator : DiscreteIntegrator  gainval=1  ExternalReset=either  SampleTime=Ts  LimitOutput=on  UpperSaturationLimit=2000  LowerSaturationLimit=-2000  ICPrevOutput=DiscIntNeverNeededParam  ICPrevScaledInput=DiscIntNeverNeededParam
  Ki : Gain  Gain=Id_Integral  SaturateOnIntegerOverflow=on  OutDataTypeStr=Inherit: Same as input  ParamDataTypeStr=Inherit: Same as input
  Kp : Gain  Gain=Id_Proportional  SaturateOnIntegerOverflow=on  OutDataTypeStr=Inherit: Same as input  ParamDataTypeStr=Inherit: Same as input
  Sum4 : Sum  SaturateOnIntegerOverflow=on
  Out : Outport
  wires:
  Ki/1 -> Discrete-Time Integrator/1
  Kp/1 -> Sum4/1
  e/1 -> Ki/1, Kp/1
  Discrete-Time Integrator/1 -> Sum4/2
  Sum4/1 -> Out/1
  RST/1 -> Discrete-Time Integrator/2
